simulink model "count_down_timer1"  (R2015b)
settings: Solver=FixedStepDiscrete  StartTime=0.0  StopTime=10.0  FixedStep=0.01  RelTol=1e-3
undefined symbols (not defined in the file): sigbuilder_block
libraries: simulink x1
settings Model: Creator=studypc2  LastModifiedBy=admin-cs
settings DataIOCC: SaveFormat=Array  SignalLogging=off
settings OptimizationCC: ExpressionDepthLimit=2147483647
settings DebuggingCC: UnderspecifiedInitializationDetection=Classic  MergeDetectMultiDrivingBlocksExec=none  SolverPrmCheckMsg=warning  StateNameClashWarn=warning
settings HardwareCC: ProdBitPerPointer=32  ProdLargestAtomicFloat=None  ProdIntDivRoundTo=Undefined  ProdEndianess=Unspecified  ProdWordSize=32  ProdHWDeviceType=32-bit Generic
settings GRTTargetCC: GeneratePreprocessorConditionals=Disable all
settings ConfigComp: CovModelRefEnable=Off

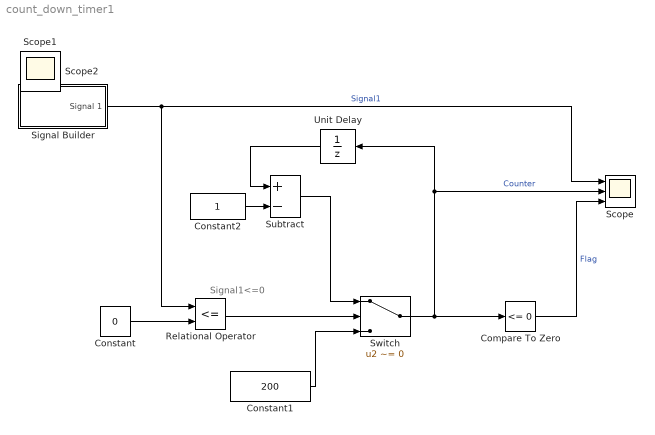
== system count_down_timer1 ==
  note: Signal1<=0
  Compare To Zero : simulink/Logic and Bit Operations/Compare To Zero  relop=<=  OutDataTypeStr=boolean
  Constant : Constant  Value=0
  Constant1 : Constant  Value=200  SampleTime=0
  Constant2 : Constant  SampleTime=0
  Relational Operator : RelationalOperator  Operator=<=  OutDataTypeStr=boolean
  Scope : Scope  NumInputPorts=3
  Signal Builder : Subsystem  Tag=STV Subsys  LoadFcn=sigbuilder_block('load');  StartFcn=sigbuilder_block('start');  StopFcn=sigbuilder_block('stop');  ClipboardFcn=sigbuilder_block('clipboard');  mask(Sigbuilder block){}
      mask help: Simulink:masks:SigbuilderBlock_MD
      mask init:
      | if ~strcmp(get_param(bdroot(gcbh),'SimulationStatus'),'stopped') tuvar = sigbuilder_block('maskInit'); end
      settings: CopyFcn=sigbuilder_block('copy');  DeleteFcn=sigbuilder_block('delete');  ModelCloseFcn=sigbuilder_block('modelClose');  PreSaveFcn=sigbuilder_block('preSave');  PauseFcn=sigbuilder_block('pause');  ContinueFcn=sigbuilder_block('continue');  NameChangeFcn=sigbuilder_block('namechange');  OpenFcn=sigbuilder_block('open',[462 109.5 550.5 393 ]);  CloseFcn=sigbuilder_block('close');
      mask Display: plot(0, 0, 100, 100,[2, 2, 32, 32, 2], [68, 8, 8, 68, 68],[32, 2], [38, 38], [32, 19, 2],[53, 60, 44], [32, 17, 17, 2],[16, 16, 31, 31]);txt = getActiveGroup(gcbh);text(2, 100, txt,'verticalAlignment', 'top');
  Subtract : Sum  Inputs=+-  OutDataTypeStr=uint16  RndMeth=Zero  SaturateOnIntegerOverflow=on
  Switch : Switch  Criteria=u2 ~= 0  RndMeth=Ceiling  SampleTime=0
  Unit Delay : UnitDelay  SampleTime=-1
  Scope1 : Scope
  Scope2 : Scope
  wires:
  Signal Builder/1(Signal 1) -> Relational Operator/1, Scope/1  "Signal1"
  Compare To Zero/1 -> Scope/3  "Flag"
  Switch/1 -> Compare To Zero/1, Scope/2, Unit Delay/1  "Counter"
  Constant1/1 -> Switch/3
  Constant/1 -> Relational Operator/2
  Relational Operator/1 -> Switch/2
  Unit Delay/1 -> Subtract/1
  Subtract/1 -> Switch/1
  Constant2/1 -> Subtract/2

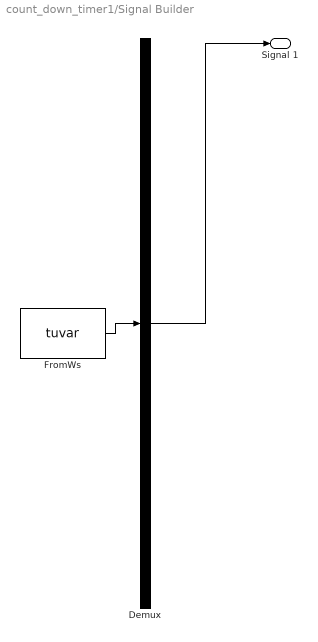
== system count_down_timer1/Signal Builder ==
  Demux : Demux  Tag=STV Demux  Outputs=1
  FromWs : FromWorkspace  Tag=STV FromWs  VariableName=tuvar  SampleTime=0
      SigBuilderData=|
      | common.afterFinalStr = 'Extrapolate'
      | common.sampleTime = 0
      | dataSet.timeRange = [0 10]
      | dataSet.name = 'Group 1'
      | sbobj.Groups.Name = 'Group 1'
      | sbobj.Groups.Signals.Name = 'Signal 1'
      | sbobj.Groups.Signals.XData = [0 2 6 10]
      | sbobj.Groups.Signals.YData = [1 0 0 0.61]
  Signal 1 : Outport  Tag=STV Outport
  wires:
  Demux/1 -> Signal 1/1
  FromWs/1 -> Demux/1
